simulink model "IEEE_14bus"  (R2021a)
settings: Solver=VariableStepAuto  StartTime=0.0  StopTime=16  RelTol=1e-3
undefined symbols (not defined in the file): c, cost, Discrete, linsys1, M, Mdot, Req, THeater, Time, TinIC
libraries: spsThreePhaseVIMeasurementLib x52, spsThreePhasePISectionLineLib x20, spsPMUPLLBasedPositiveSequenceLib x14, spsThreePhaseSeriesRLCLoadLib x12, spsThreePhaseTransformerTwoWindingsLib x6, simulink x6, spsThreePhaseBreakerLib x4, rllib x3, simulink_extras x3, eeStairGenerator x3, spsThreePhaseSourceLib x3, spsSynchronousMachinepuStandardLib x3
(part 1 of 3)
settings Model: Creator=User  LastModifiedBy=hpirc
settings DataIOCC: SaveFinalState=on  SaveOperatingPoint=on

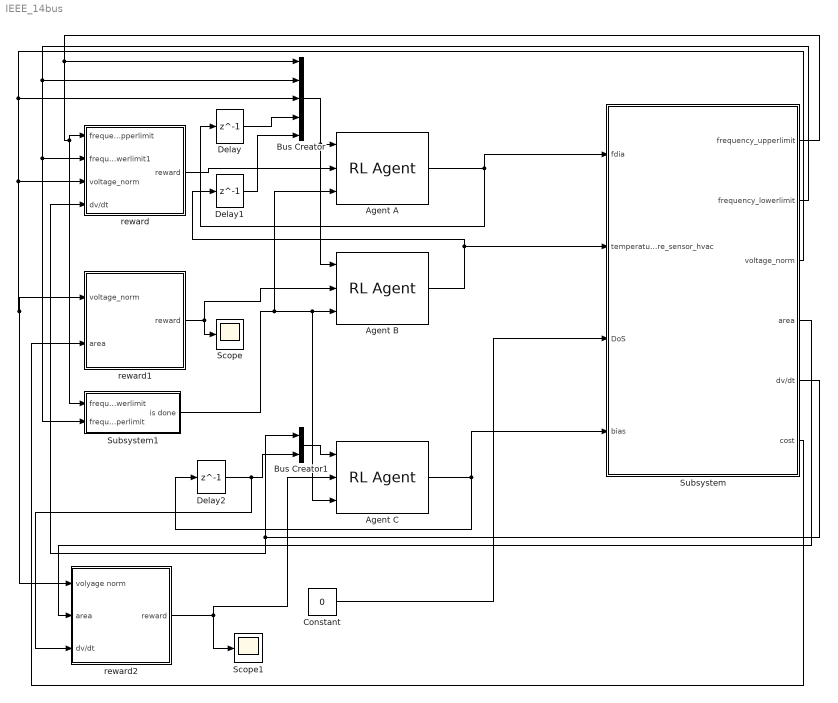
== system IEEE_14bus ==
  Agent A : rllib/RL Agent  Agent=agent1  ExternalActionAsInput=off  ProvideCumRwd=off  TreatAsDirectFeedthrough=on
  Agent B : rllib/RL Agent  Agent=agent2  ExternalActionAsInput=off  ProvideCumRwd=off  TreatAsDirectFeedthrough=on
  Agent C : rllib/RL Agent  Agent=agent3  ExternalActionAsInput=off  ProvideCumRwd=off  TreatAsDirectFeedthrough=on
  Bus Creator : BusCreator  Inputs=5
  Bus Creator1 : BusCreator  Inputs=2
  Constant : Constant  Value=0
  Delay : Delay  DelayLength=1  InputProcessing=Columns as channels (frame based)
  Delay1 : Delay  DelayLength=1  InputProcessing=Columns as channels (frame based)
  Delay2 : Delay  DelayLength=1  InputProcessing=Columns as channels (frame based)
  Scope : Scope
  Scope1 : Scope
  Subsystem : Subsystem
  Subsystem1 : Subsystem
  reward : Subsystem
  reward1 : Subsystem
  reward2 : Subsystem
  wires:
  Agent A/1 -> Delay/1, Subsystem/1(fdia)
  Agent B/1 -> Delay1/1, Subsystem/2(temperature_sensor_hvac)
  Constant/1 -> Subsystem/3(DoS)
  reward/1(reward) -> Agent A/2
  Subsystem/1(frequency_upperlimit) -> Subsystem1/1(frequency_lowerlimit), reward/1(frequency_upperlimit), Bus Creator/1
  Subsystem/2(frequency_lowerlimit) -> Subsystem1/2(frequency_upperlimit), reward/2(frequency_lowerlimit1), Bus Creator/2
  Subsystem/3(voltage_norm) -> reward2/1(volyage norm), reward1/1(voltage_norm), reward/3(voltage_norm), Bus Creator/3
  Delay/1 -> Bus Creator/4
  Bus Creator/1 -> Agent B/1, Agent A/1
  Subsystem/4(area) -> reward2/2(area)
  reward1/1(reward) -> Agent B/2, Scope/1
  Subsystem1/1(is done) -> Agent A/3, Agent C/3, Agent B/3
  Delay1/1 -> Bus Creator/5
  Agent C/1 -> Subsystem/4(bias), Delay2/1
  Subsystem/5(dv/dt) -> Bus Creator1/1, reward/4(dv/dt)
  Delay2/1 -> reward2/3(dv/dt), Bus Creator1/2
  Bus Creator1/1 -> Agent C/1
  reward2/1(reward) -> Agent C/2, Scope1/1
  Subsystem/6(cost) -> reward1/2(area)
